simulink model "fuzzy_final"  (R2015b)
settings: Solver=VariableStepAuto  StartTime=0.0  StopTime=10  RelTol=1e-3
undefined symbols (not defined in the file): flc
libraries: powerlib x24, fuzblock x1, re_lib x1, simulink x1
settings Model: Creator=SPIRO  LastModifiedBy=SPIRO-POWER
settings SolverCC: AlgebraicLoopSolver=LineSearch

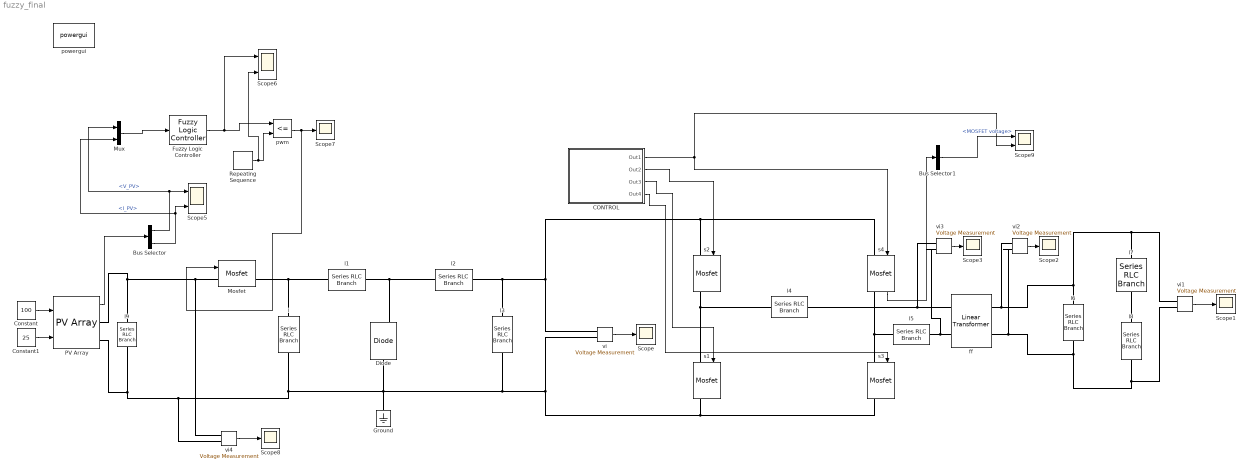
== system fuzzy_final ==
  Bus Selector : BusSelector  OutputSignals=V_PV,I_PV
  Bus Selector1 : BusSelector  OutputSignals=MOSFET voltage
  CONTROL : Subsystem
  Constant : Constant  Value=100
  Constant1 : Constant  Value=25
  Diode : powerlib/Power Electronics/Diode  Ron=0.001  Lon=0  Vf=0.8  IC=0  UseSnubber=off  Rs=500  Cs=250e-9  Measurements=on
  Fuzzy Logic Controller : fuzblock/Fuzzy Logic  Controller  fis=[flc]
  Ground : powerlib/Elements/Ground  LConnTagsString=a
  Mosfet : powerlib/Power Electronics/Mosfet  Ron=0.1  Lon=0  Rd=0.01  Vfd=0  IC=0  Rs=1e5  Cs=inf  Measurements=on
  Mux : Mux  Inputs=2
  PV Array : re_lib/Solar/PV Array  Npar=40  Nser=10  PlotType=array @ 1000 W/m2 & specified temperatures  S_vec="[ 1000  500  100 ]"  Temp_C_vec="[ 45 25  ]"  ModuleName=1Soltech 1STH-215-P  PlotWhenSelected=off  Pm=213.15  Ncell=60  Voc=36.3  Isc=7.84  Vm=29  Im=7.35  beta_Voc_pc=-0.36099  alpha_Isc_pc=0.102  beta_Voc=-0.13104  alpha_Isc=0.007997  IL=7.8649  I0=2.9259e-10  nI=0.98117  Rsh=313.3991  Rs=0.39383  BAL=off  Tc=1e-6  Tfilter=5e-5
  Repeating Sequence : simulink/Sources/Repeating Sequence  rep_seq_t=[0 .0001 .0002]  rep_seq_y=[0 2 0]
  Scope{,1..3,7..8} (6 alike) : Scope
  Scope5 : Scope  NumInputPorts=2
  Scope6 : Scope  NumInputPorts=2
  Scope9 : Scope  NumInputPorts=2
  ff : powerlib/Elements/Linear Transformer  UNITS=pu  NominalPower=[ 250e3 50 ]  winding1="[ 1500  0.02  0.8 ]"  winding2="[ 2000  0.02  0.8 ]"  ThreeWindings=off  winding3=[ 315e3 0.002 0.08 ]  RmLm=[ 10 25]  Measurements=None  DataType=off
  l : powerlib/Elements/Series RLC Branch  LConnTagsString=__new0  RConnTagsString=__new0  BranchType=L  Resistance=1  Inductance=10  SetiL0=off  InitialCurrent=0  Capacitance=1e-6  Setx0=off  InitialVoltage=0  Measurements=None
  l1 : powerlib/Elements/Series RLC Branch  LConnTagsString=__new0  RConnTagsString=__new0  BranchType=C  Resistance=1  Inductance=1e-3  SetiL0=off  InitialCurrent=0  Capacitance=2e-4  Setx0=off  InitialVoltage=0  Measurements=None
  l2 : powerlib/Elements/Series RLC Branch  LConnTagsString=__new0  RConnTagsString=__new0  BranchType=L  Resistance=1  Inductance=20  SetiL0=off  InitialCurrent=0  Capacitance=1e-6  Setx0=off  InitialVoltage=0  Measurements=None
  l3 : powerlib/Elements/Series RLC Branch  LConnTagsString=__new0  RConnTagsString=__new0  BranchType=C  Resistance=1  Inductance=1e-3  SetiL0=off  InitialCurrent=0  Capacitance=5000e-6  Setx0=off  InitialVoltage=0  Measurements=None
  l4 : powerlib/Elements/Series RLC Branch  LConnTagsString=__new0  RConnTagsString=__new0  BranchType=L  Resistance=1  Inductance=20e-6  SetiL0=off  InitialCurrent=0  Capacitance=1e-6  Setx0=off  InitialVoltage=0  Measurements=None
  l5 : powerlib/Elements/Series RLC Branch  LConnTagsString=__new0  RConnTagsString=__new0  BranchType=C  Resistance=1  Inductance=20  SetiL0=off  InitialCurrent=0  Capacitance=1000e-5  Setx0=off  InitialVoltage=0  Measurements=None
  l6 : powerlib/Elements/Series RLC Branch  LConnTagsString=__new0  RConnTagsString=__new0  BranchType=C  Resistance=1  Inductance=20  SetiL0=off  InitialCurrent=0  Capacitance=100e-6  Setx0=off  InitialVoltage=0  Measurements=None
  l7 : powerlib/Elements/Series RLC Branch  LConnTagsString=__new0  RConnTagsString=__new0  BranchType=L  Resistance=1  Inductance=20e-2  SetiL0=off  InitialCurrent=0  Capacitance=1e-6  Setx0=off  InitialVoltage=0  Measurements=None
  l8 : powerlib/Elements/Series RLC Branch  LConnTagsString=__new0  RConnTagsString=__new0  BranchType=R  Resistance=10  Inductance=20  SetiL0=off  InitialCurrent=0  Capacitance=1e-6  Setx0=off  InitialVoltage=0  Measurements=None
  l9 : powerlib/Elements/Series RLC Branch  LConnTagsString=__new0  RConnTagsString=__new0  BranchType=C  Resistance=1  Inductance=1e-3  SetiL0=off  InitialCurrent=0  Capacitance=2e-4  Setx0=off  InitialVoltage=0  Measurements=None
  powergui : powerlib/powergui  Priority=1  SimulationMode=Discrete  SolverType=Tustin/Backward Euler (TBE)  SampleTime=50e-6  frequency=60  SPID=off  DisableSnubberDevices=off  DisableRonSwitches=off  DisableVfSwitches=off  SwTol=0  DisplayEquations=off  Interpol=off  ExternalGateDelay=off  methode=off  Ts=10  FunctionMessages=off  echomessages=off  HookPort=off  EnableUseOfTLC=off  x0status=blocks  frequencyindice=0  Pbase=100e6  ErrMax=1e-4  Iterations=50  UnitsV=kV  UnitsW=MW  buscounter=0  RestoreLinks=warning  ResistiveCurrentMeasurement=off  Frange=[0:2:500]  Ylog=off  Xlog=on  ShowGrid=off  save=off  variable=ZData  structure=0  ZoomFFT=off  StartTime=0.0  cycles=1  DisplayStyle=1  fundamental=60  FreqAxis=off  MaxFrequency=1000  frequencyindicesteady=1  RmsSteady=1  display=off
  pwm : RelationalOperator  Operator=<=  OutDataTypeStr=boolean
  s{1..4} (4 alike) : powerlib/Power Electronics/Mosfet  Ron=0.1  Lon=0  Rd=0.01  Vfd=0  IC=0  Rs=1e5  Cs=inf  Measurements=on
  vi{,1..4} (5 alike) : powerlib/Measurements/Voltage Measurement  PhasorSimulation=off  OutputType=Complex  PSBequivalent=0
  wires:
  pwm/1 -> Mosfet/1, Scope7/1
  vi/1 -> Scope/1
  vi1/1 -> Scope1/1
  vi2/1 -> Scope2/1
  vi3/1 -> Scope3/1
  Constant/1 -> PV Array/1
  Constant1/1 -> PV Array/2
  PV Array/1 -> Bus Selector/1
  Bus Selector/1 -> Scope5/1, Mux/1  "<V_PV>"
  Bus Selector/2 -> Mux/2, Scope5/2  "<I_PV>"
  Mux/1 -> Fuzzy Logic Controller/1
  Fuzzy Logic Controller/1 -> Scope6/1, pwm/1
  Repeating Sequence/1 -> Scope6/2, pwm/2
  vi4/1 -> Scope8/1
  s4/1 -> Bus Selector1/1
  Bus Selector1/1 -> Scope9/1  "<MOSFET voltage>"
  CONTROL/1(Out1) -> Scope9/2, s4/1
  CONTROL/2(Out2) -> s2/1
  CONTROL/3(Out3) -> s1/1
  CONTROL/4(Out4) -> s3/1
  connections:
  Mosfet/LConn1 -- vi4/LConn1 -- PV Array/RConn1 -- l9/LConn1
  Mosfet/RConn1 -- l/LConn1 -- l1/RConn1
  l2/RConn1 -- Diode/RConn1 -- l1/LConn1
  s2/RConn1 -- s1/LConn1 -- l4/RConn1
  s4/RConn1 -- l5/RConn1 -- s3/LConn1
  l4/LConn1 -- vi3/LConn1 -- ff/LConn1
  l5/LConn1 -- vi3/LConn2 -- ff/LConn2
  l8/LConn1 -- l7/RConn1
  l6/LConn1 -- vi2/LConn1 -- ff/RConn1 -- vi1/LConn1 -- l7/LConn1
  l6/RConn1 -- vi2/LConn2 -- ff/RConn2 -- vi1/LConn2 -- l8/RConn1
  l3/LConn1 -- vi/LConn1 -- s2/LConn1 -- s4/LConn1 -- l2/LConn1
  vi4/LConn2 -- l9/RConn1 -- PV Array/RConn2 -- l/RConn1 -- Ground/LConn1 -- Diode/LConn1 -- vi/LConn2 -- s3/RConn1 -- s1/RConn1 -- l3/RConn1

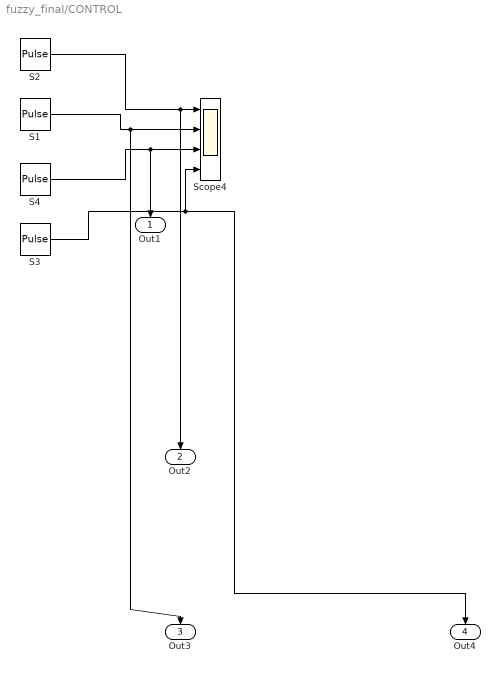
== system fuzzy_final/CONTROL ==
  S1 : DiscretePulseGenerator  PulseType=Time based  Period=.02  PulseWidth=45  PhaseDelay=(55/100)*.02
  S2 : DiscretePulseGenerator  PulseType=Time based  Period=.02  PulseWidth=50
  S3 : DiscretePulseGenerator  PulseType=Time based  Period=.02  PulseWidth=(1.5/6)*100
  S4 : DiscretePulseGenerator  PulseType=Time based  Period=.02  PulseWidth=(4/6)*100  PhaseDelay=(2/6)*.02
  Scope4 : Scope  NumInputPorts=4
  Out1 : Outport
  Out2 : Outport  Port=2
  Out3 : Outport  Port=3
  Out4 : Outport  Port=4
  wires:
  S2/1 -> Out2/1, Scope4/1
  S4/1 -> Out1/1, Scope4/3
  S1/1 -> Scope4/2, Out3/1
  S3/1 -> Out4/1, Scope4/4
